simulink model "mpc"  (R2023b)
settings: Solver=FixedStepAuto  StartTime=0.0  StopTime=t_max  FixedStep=dt_max  RelTol=1e-3
values from neighbouring files (symbols this model uses):
  dt_max = 0.01    [UR5_Details.m]    (also in mpc_script.m; smc.m)
  m = 3    [mpc_script.m]    (also in smc.m = 7)
  n = 3    [mpc_script.m]    (also in smc.m)
  p = 10    [mpc_script.m]    (also in smc.m = 5)
  theta_0 = zeros(n,1)    [mpc_script.m]    (also in smc.m)
  theta_dot0 = zeros(n,1)    [mpc_script.m]    (also in smc.m)
undefined symbols (not defined in the file or in its folder): Np, u_0
libraries: simulink x3
settings Model: Creator=dimitriasilveria  LastModifiedBy=sham_
settings OptimizationCC: ReuseModelBlockBuffer=off

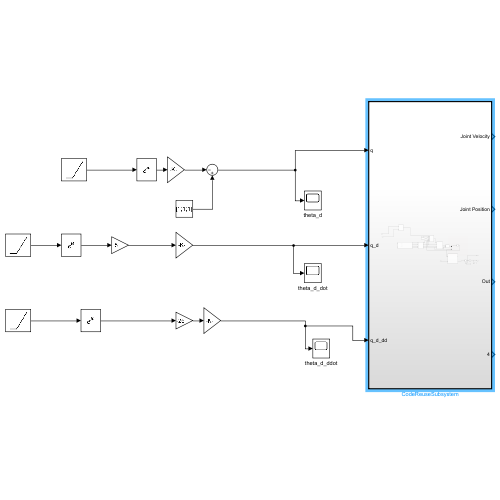
[thumbnail: Simulink's stored preview of the top-level diagram]
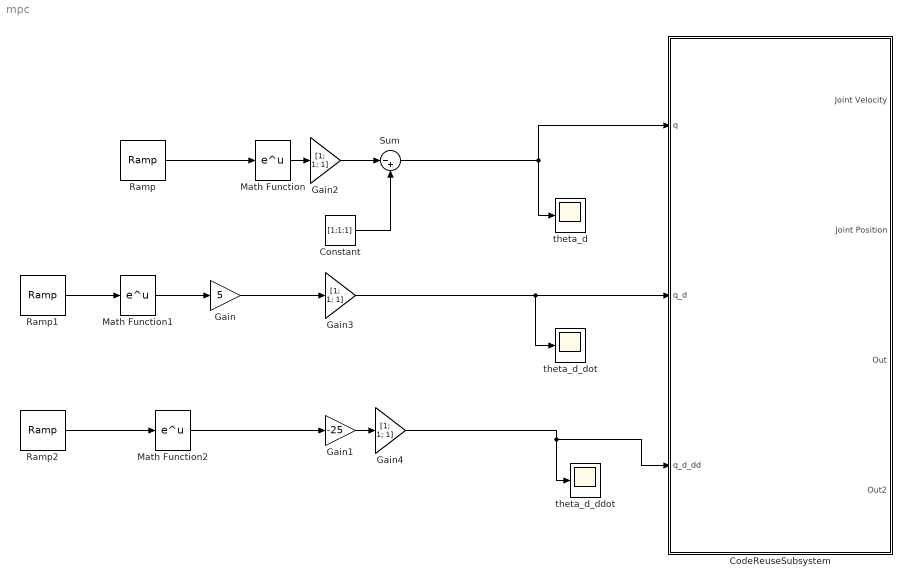
== system mpc ==
  CodeReuseSubsystem : Subsystem  TreatAsAtomicUnit=on
      settings: RTWFcnNameOpts=Use subsystem name  RTWFileNameOpts=Use function name
  Constant : Constant  Value=[1;1;1]
  Gain : Gain  Gain=5
  Gain1 : Gain  Gain=-25
  Gain2 : Gain  Gain=[1; 1; 1]
  Gain3 : Gain  Gain=[1; 1; 1]
  Gain4 : Gain  Gain=[1; 1; 1]
  Math Function : Math
  Math Function1 : Math
  Math Function2 : Math
  Ramp : simulink/Sources/Ramp  slope=-5  start=0  InitialOutput=0
  Ramp1 : simulink/Sources/Ramp  slope=-5  start=0  InitialOutput=0
  Ramp2 : simulink/Sources/Ramp  slope=-5  start=0  InitialOutput=0
  Sum : Sum  Inputs=|-+
  theta_d : Scope
  theta_d_ddot : Scope
  theta_d_dot : Scope
  wires:
  Gain4/1 -> CodeReuseSubsystem/3(q_d_dd), theta_d_ddot/1
  Gain2/1 -> Sum/1
  Constant/1 -> Sum/2
  Math Function/1 -> Gain2/1
  Ramp/1 -> Math Function/1
  Math Function1/1 -> Gain/1
  Gain3/1 -> CodeReuseSubsystem/2(q_d), theta_d_dot/1
  Math Function2/1 -> Gain1/1
  Ramp1/1 -> Math Function1/1
  Ramp2/1 -> Math Function2/1
  Sum/1 -> CodeReuseSubsystem/1(q), theta_d/1
  Gain/1 -> Gain3/1
  Gain1/1 -> Gain4/1

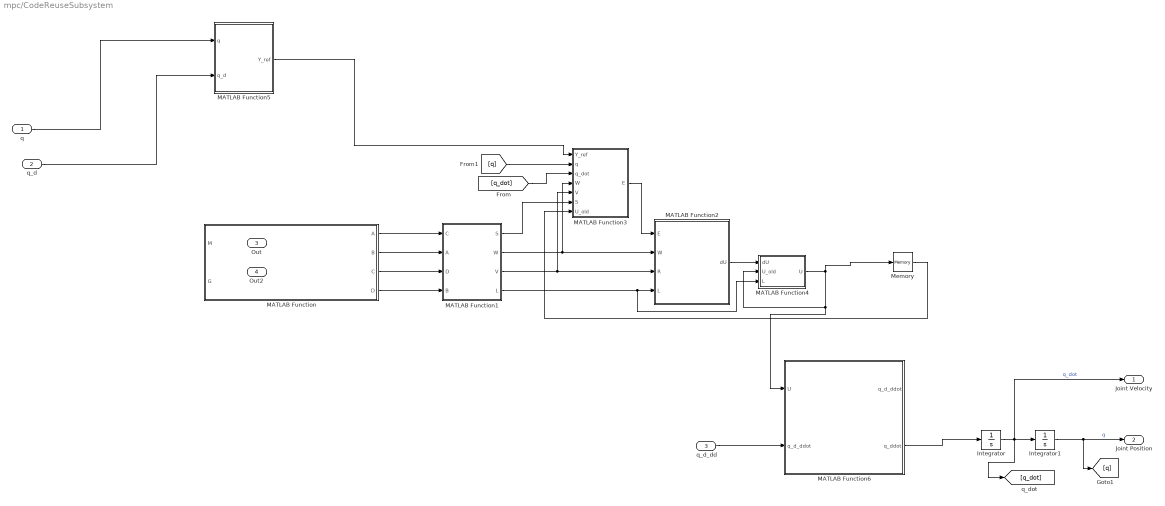
== system mpc/CodeReuseSubsystem ==
  q : Inport
  q_d : Inport  Port=2
  q_d_dd : Inport  Port=3
  Integrator : Integrator  InitialCondition=theta_dot0
  Integrator1 : Integrator  InitialCondition=theta_0
  MATLAB Function : MATLAB Function  TreatAsAtomicUnit=on
  MATLAB Function1 : MATLAB Function  TreatAsAtomicUnit=on
  MATLAB Function2 : MATLAB Function  TreatAsAtomicUnit=on
  MATLAB Function3 : MATLAB Function  TreatAsAtomicUnit=on
  MATLAB Function4 : MATLAB Function  TreatAsAtomicUnit=on
  MATLAB Function5 : MATLAB Function  TreatAsAtomicUnit=on
  MATLAB Function6 : MATLAB Function  TreatAsAtomicUnit=on
  Memory : Memory  InitialCondition=u_0  InheritSampleTime=on
  Joint Velocity : Outport  Unit=rad/s
  Joint Position : Outport  Port=2  Unit=rad
  Out : Outport  Port=3
  Out2 : Outport  Port=4
  wires:
  MATLAB Function1/3(V) -> MATLAB Function3/5(V), MATLAB Function2/3(R)
  MATLAB Function1/4(L) -> MATLAB Function4/3(L), MATLAB Function2/4(L)
  MATLAB Function4/1(U) -> Memory/1, MATLAB Function6/1(U), MATLAB Function4/2(U_old)
  MATLAB Function/4(D) -> MATLAB Function1/4(B)
  MATLAB Function/2(B) -> MATLAB Function1/2(A)
  MATLAB Function/3(C) -> MATLAB Function1/3(D)
  MATLAB Function/1(A) -> MATLAB Function1/1(C)
  MATLAB Function1/2(W) -> MATLAB Function3/4(W), MATLAB Function2/2(W)
  MATLAB Function1/1(S) -> MATLAB Function3/6(S)
  Memory/1 -> MATLAB Function3/7(U_old)
  MATLAB Function2/1(dU) -> MATLAB Function4/1(dU)
  MATLAB Function3/1(E) -> MATLAB Function2/1(E)
  q/1 -> MATLAB Function5/1(q)
  q_d/1 -> MATLAB Function5/2(q_d)
  MATLAB Function5/1(Y_ref) -> MATLAB Function3/1(Y_ref)
  Integrator/1 -> [q_dot], Joint Velocity/1, Integrator1/1  "q_dot"
  Integrator1/1 -> [q], Joint Position/1  "q"
  MATLAB Function6/2(q_ddot) -> Integrator/1
  [q] -> MATLAB Function3/2(q)
  [q_dot] -> MATLAB Function3/3(q_dot)
  q_d_dd/1 -> MATLAB Function6/2("q_d_ddot ")

== matlab function mpc/CodeReuseSubsystem/MATLAB Function1 ==
  data: S output; W output; V output; L output; p parameter; m parameter; Np parameter; C input; A input; D input; B input
function [S,W,V,L] = matrices(p, m, Np,C,A,D,B)
%Np = P*dt_max;
%Nm = m*d_t_max;
S = [];
W = [];
V = [];
L = [];
L1 = [];
L2 = [];

for i = 1:Np
    S = [S;C*A.^i];
end
l_v = C*D*0;
k = p;
for i = 1:p
   if i < p
       L1 = [L1;eye(n)];
   else:
       L1 = [L1;zeros(n)];
   end
   L2 = [L2;eye(n)];
   l_v = l_v + C*A.^(Np-k)*D;
   V = [V;l_v];   
   k = k - 1;
   l = [];
   for j = 1:p
       if j<=i
           l = [l C*A.^(i-j)*B];
       else
           l = [l 0*C*A*B];
       end
  W = [W;l];
    end
end
for i=1:m
    if i == 1
        L = [L1];
    else:
        L = [L;L2];
    end

end

== matlab function mpc/CodeReuseSubsystem/MATLAB Function ==
  data: A output; M input; G input; B output; C output; D output; n parameter; dt_max parameter
function [A,B,C,D] = state_space_matrices(M,G, n, dt_max)
%n is the number of joints 
I_n = eye(n);
O_n = zeros(n);
k = inv(M);
A = [I_n dt_max*I_n;O_n I_n];
B = [(dt_max^2/2)*k;dt_max*k];
C = [I_n O_n];
g = -inv(M)*C + G; %here I am also assuming C = C(q,q_dot)*q_dot

D = [(dt_max^2/2)*g;dt_max*g];

== matlab function mpc/CodeReuseSubsystem/MATLAB Function2 ==
  data: E input; W input; R input; L input; dU output; Q parameter
function dU = optimization(E,W,R,L, Q)
H = 0.5*(L'*W'*Q'*Q*W*L + R'*R);
f = -2*L'*W'*Q'*Q*E;

dU = quadprog(H,f);

== matlab function mpc/CodeReuseSubsystem/MATLAB Function3 ==
  data: Y_ref input; q input; q_dot input; W input; V input; E output; S input; U_old input
function E = error(Y_ref,q,q_dot,W,V,S,U_old)
%Y_ref and q_d are the same person
x = [q;q_dot];
E = Y_ref - S*x - W*U_old - V;

== matlab function mpc/CodeReuseSubsystem/MATLAB Function4 ==
  data: dU input; U output; U_old input; L input
function U = input(dU,U_old,L)
    U = U_old + L*dU;

== matlab function mpc/CodeReuseSubsystem/MATLAB Function5 ==
  data: q input; Y_ref output; q_d input
function Y_ref = fcn(q,q_d)

Y_ref = [q;q_d];

== matlab function mpc/CodeReuseSubsystem/MATLAB Function6 ==
  data: U input; q_d_ddot output; q_ddot output; q_d_ddot input
function [q_d_ddot,q_ddot] = fcn(U,q_d_ddot)

q_ddot = q_d_ddot;
